simulink model "ALS_Project"  (R2020a)
settings: Solver=FixedStepDiscrete  StartTime=0.0  StopTime=10.0  FixedStep=1  RelTol=1e-3
values from neighbouring files (symbols this model uses):
  Als_mode : value not decoded    [ALS_Project_dd.sldd]
  Carangle = 25.0    [ALS_Project_dd.sldd]    (also in Car_Angle.m = Simulink.Parameter)
  Door_locks : value not decoded    [ALS_Project_dd.sldd]
  Ignition : value not decoded    [ALS_Project_dd.sldd]
  Lanes : value not decoded    [ALS_Project_dd.sldd]
  Lights : value not decoded    [ALS_Project_dd.sldd]
  Obstacles : value not decoded    [ALS_Project_dd.sldd]
  Roads : value not decoded    [ALS_Project_dd.sldd]
  Time = 2.0    [ALS_Project_dd.sldd]    (also in Car_Angle.m = Simulink.Parameter)
  Tunnel : value not decoded    [ALS_Project_dd.sldd]
  Visual : value not decoded    [ALS_Project_dd.sldd]
  Weather : value not decoded    [ALS_Project_dd.sldd]
libraries: simulink x53
settings Model: Creator=hp  LastModifiedBy=hp

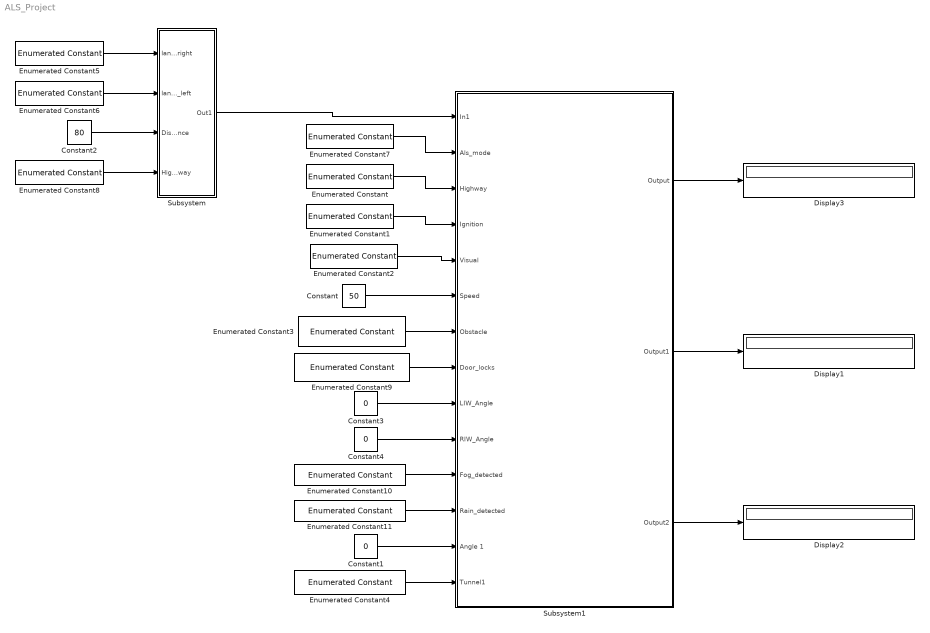
== system ALS_Project ==
  Constant : Constant  Value=50
  Constant1 : Constant  Value=0
  Constant2 : Constant  Value=80
  Constant3 : Constant  Value=0
  Constant4 : Constant  Value=0
  Display1 : Display
  Display2 : Display
  Display3 : Display
  Enumerated Constant : simulink/Sources/Enumerated Constant  OutDataTypeStr=Enum:Roads  Value=Roads.City_road  SampleTime=inf
  Enumerated Constant1 : simulink/Sources/Enumerated Constant  OutDataTypeStr=Enum: Ignition  Value=Ignition.Off  SampleTime=inf
  Enumerated Constant10 : simulink/Sources/Enumerated Constant  OutDataTypeStr=Enum: Weather  Value=Weather.Fog_detected  SampleTime=inf
  Enumerated Constant11 : simulink/Sources/Enumerated Constant  OutDataTypeStr=Enum: Weather  Value=Weather.Rain_detected  SampleTime=inf
  Enumerated Constant2 : simulink/Sources/Enumerated Constant  OutDataTypeStr=Enum: Visual  Value=Visual.Night_mode  SampleTime=inf
  Enumerated Constant3 : simulink/Sources/Enumerated Constant  OutDataTypeStr=Enum: Obstacles  Value=Obstacles.No_Obstacle_detected  SampleTime=inf
  Enumerated Constant4 : simulink/Sources/Enumerated Constant  OutDataTypeStr=Enum: Tunnel  Value=Tunnel.No_Tunnel_detected  SampleTime=inf
  Enumerated Constant5 : simulink/Sources/Enumerated Constant  OutDataTypeStr=Enum: Lanes  Value=Lanes.Lane3_right  SampleTime=inf
  Enumerated Constant6 : simulink/Sources/Enumerated Constant  OutDataTypeStr=Enum: Lanes  Value=Lanes.NoVehicle  SampleTime=inf
  Enumerated Constant7 : simulink/Sources/Enumerated Constant  OutDataTypeStr=Enum: Als_mode  Value=Als_mode.enable  SampleTime=inf
  Enumerated Constant8 : simulink/Sources/Enumerated Constant  OutDataTypeStr=Enum:Roads  Value=Roads.Highway  SampleTime=inf
  Enumerated Constant9 : simulink/Sources/Enumerated Constant  OutDataTypeStr=Enum: Door_locks  Value=Door_locks.Door_locked  SampleTime=inf
  Subsystem : Subsystem  Description=describes about the lanes scenario
  Subsystem1 : Subsystem  Description=normal lightening on highway
  wires:
  Subsystem/1(Out1) -> Subsystem1/1(In1)
  Enumerated Constant/1 -> Subsystem1/3(Highway)
  Enumerated Constant1/1 -> Subsystem1/4(Ignition)
  Enumerated Constant2/1 -> Subsystem1/5(Visual)
  Constant/1 -> Subsystem1/6(Speed)
  Enumerated Constant3/1 -> Subsystem1/7(Obstacle)
  Constant2/1 -> Subsystem/3(Distance)
  Enumerated Constant5/1 -> Subsystem/1(lane1_right)
  Enumerated Constant6/1 -> Subsystem/2(lane1_left)
  Enumerated Constant7/1 -> Subsystem1/2(Als_mode)
  Enumerated Constant8/1 -> Subsystem/4(Highway)
  Enumerated Constant9/1 -> Subsystem1/8(Door_locks)
  Constant4/1 -> Subsystem1/10(RIW_Angle)
  Constant3/1 -> Subsystem1/9(LIW_Angle)
  Constant1/1 -> Subsystem1/13(Angle 1)
  Enumerated Constant4/1 -> Subsystem1/14(Tunnel1)
  Subsystem1/3(Output2) -> Display2/1
  Subsystem1/2(Output1) -> Display1/1
  Subsystem1/1(Output) -> Display3/1
  Enumerated Constant11/1 -> Subsystem1/12(Rain_detected)
  Enumerated Constant10/1 -> Subsystem1/11(Fog_detected)

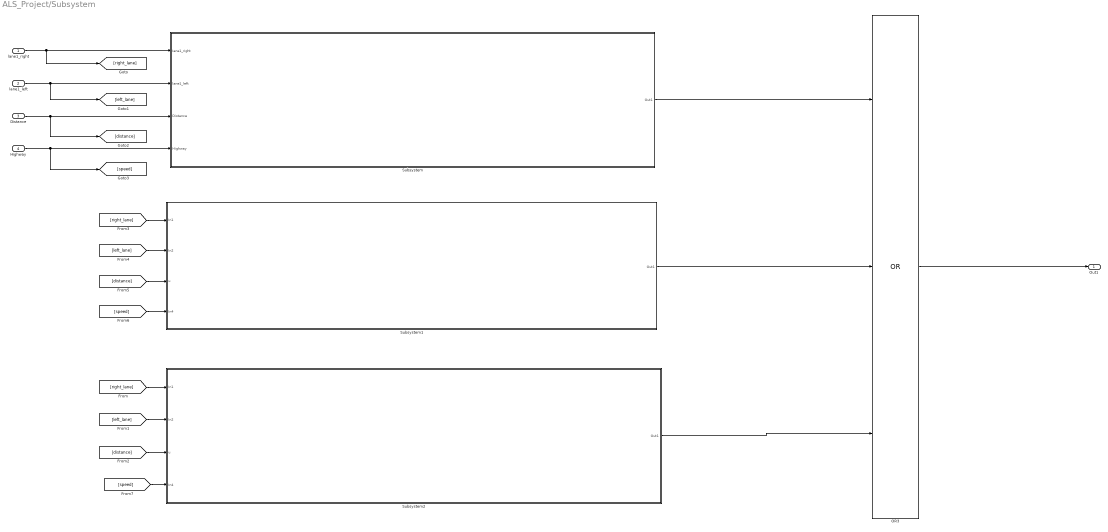
== system ALS_Project/Subsystem ==
  lane1_right : Inport
  lane1_left : Inport  Port=2
  Distance : Inport  Port=3
  Highway : Inport  Port=4
  OR3 : Logic  Operator=OR  Inputs=3  AllPortsSameDT=off  OutDataTypeStr=boolean
  Subsystem : Subsystem  Description=describes about the lane1 scenario
  Subsystem1 : Subsystem  Description=describes about the lane2 scenario
  Subsystem2 : Subsystem  Description=describes about the lane3 scenario
  Out1 : Outport
  wires:
  Highway/1 -> [speed], Subsystem/4(Highway)
  Subsystem1/1(Out1) -> OR3/2
  Subsystem/1(Out1) -> OR3/1
  Subsystem2/1(Out1) -> OR3/3
  lane1_left/1 -> [left_lane], Subsystem/2(lane1_left)
  Distance/1 -> [distance], Subsystem/3(Distance)
  lane1_right/1 -> [right_lane], Subsystem/1(Iane1_right)
  OR3/1 -> Out1/1
  [right_lane] -> Subsystem2/1(In1)
  [left_lane] -> Subsystem2/2(In2)
  [right_lane] -> Subsystem1/1(In1)
  [left_lane] -> Subsystem1/2(In2)
  [distance] -> Subsystem2/3(u)
  [distance] -> Subsystem1/3(u)
  [speed] -> Subsystem1/4(In4)
  [speed] -> Subsystem2/4(In4)

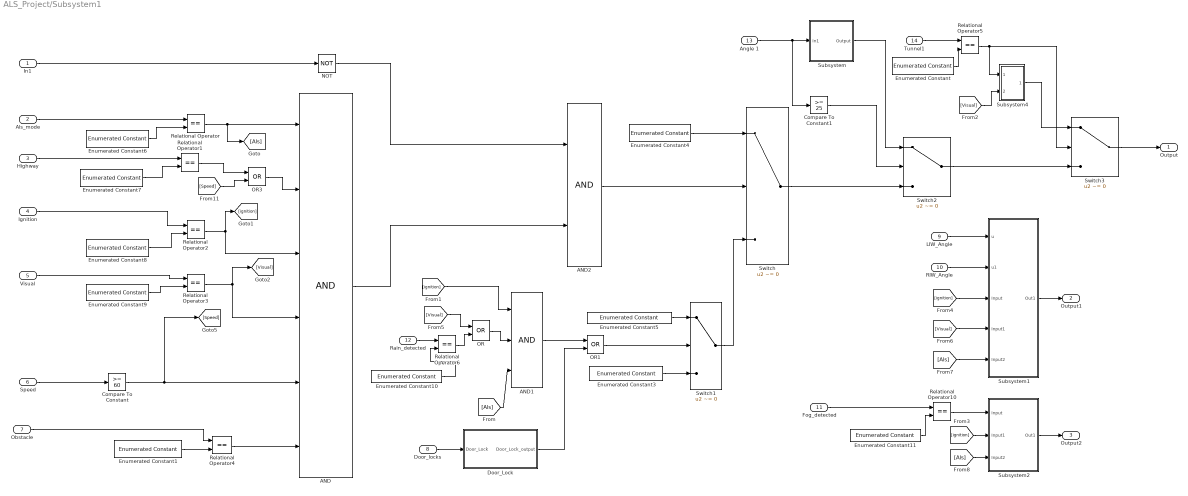
== system ALS_Project/Subsystem1 ==
  In1 : Inport
  Als_mode : Inport  Port=2
  Highway : Inport  Port=3
  Ignition : Inport  Port=4
  Visual : Inport  Port=5
  Speed : Inport  Port=6
  Obstacle : Inport  Port=7
  Door_locks : Inport  Port=8
  LIW_Angle : Inport  Port=9
  RIW_Angle : Inport  Port=10
  Fog_detected : Inport  Port=11
  Rain_detected : Inport  Port=12
  Angle 1 : Inport  Port=13
  Tunnel1 : Inport  Port=14
  AND : Logic  Inputs=6  AllPortsSameDT=off  OutDataTypeStr=boolean
  AND1 : Logic  Inputs=3  AllPortsSameDT=off  OutDataTypeStr=boolean
  AND2 : Logic  AllPortsSameDT=off  OutDataTypeStr=boolean
  Compare To Constant : simulink/Logic and Bit Operations/Compare To Constant  relop=>=  const=60  OutDataTypeStr=boolean
  Compare To Constant1 : simulink/Logic and Bit Operations/Compare To Constant  relop=>=  const=25  OutDataTypeStr=boolean
  Door_Lock : Subsystem
  Enumerated Constant : simulink/Sources/Enumerated Constant  OutDataTypeStr=Enum: Tunnel  Value=Tunnel.Tunnel_detected  SampleTime=inf
  Enumerated Constant1 : simulink/Sources/Enumerated Constant  OutDataTypeStr=Enum:Obstacles  Value=Obstacles.No_Obstacle_detected  SampleTime=inf
  Enumerated Constant10 : simulink/Sources/Enumerated Constant  OutDataTypeStr=Enum: Weather  Value=Weather.Rain_detected  SampleTime=inf
  Enumerated Constant11 : simulink/Sources/Enumerated Constant  OutDataTypeStr=Enum: Weather  Value=Weather.Fog_detected  SampleTime=inf
  Enumerated Constant3 : simulink/Sources/Enumerated Constant  OutDataTypeStr=Enum: Lights  Value=Lights.Headlights_Off  SampleTime=inf
  Enumerated Constant4 : simulink/Sources/Enumerated Constant  OutDataTypeStr=Enum: Lights  Value=Lights.High_Beam  SampleTime=inf
  Enumerated Constant5 : simulink/Sources/Enumerated Constant  OutDataTypeStr=Enum: Lights  Value=Lights.Low_Beam  SampleTime=inf
  Enumerated Constant6 : simulink/Sources/Enumerated Constant  OutDataTypeStr=Enum: Als_mode  Value=Als_mode.enable  SampleTime=inf
  Enumerated Constant7 : simulink/Sources/Enumerated Constant  OutDataTypeStr=Enum: Roads  Value=Roads.Highway  SampleTime=inf
  Enumerated Constant8 : simulink/Sources/Enumerated Constant  OutDataTypeStr=Enum: Ignition  Value=Ignition.On  SampleTime=inf
  Enumerated Constant9 : simulink/Sources/Enumerated Constant  OutDataTypeStr=Enum: Visual  Value=Visual.Night_mode  SampleTime=inf
  NOT : Logic  Operator=NOT  IconShape=distinctive  AllPortsSameDT=off  OutDataTypeStr=boolean
  OR : Logic  Operator=OR  AllPortsSameDT=off  OutDataTypeStr=boolean
  OR1 : Logic  Operator=OR  AllPortsSameDT=off  OutDataTypeStr=boolean
  OR3 : Logic  Operator=OR  AllPortsSameDT=off  OutDataTypeStr=boolean
  Relational Operator{,1..6,10} (8 alike) : RelationalOperator  Operator===  OutDataTypeStr=boolean  RndMeth=Simplest
  Subsystem : Subsystem
  Subsystem1 : Subsystem
  Subsystem2 : Subsystem
  Subsystem4 : Subsystem
  Switch{,1..3} (4 alike) : Switch  Criteria=u2 ~= 0
  Output : Outport
  Output1 : Outport  Port=2
  Output2 : Outport  Port=3
  wires:
  Relational Operator3/1 -> [Visual], AND/4
  Relational Operator/1 -> [Als], AND/1
  Relational Operator2/1 -> [ignition], AND/3
  Enumerated Constant7/1 -> Relational Operator1/2
  Switch1/1 -> Switch/3
  Enumerated Constant9/1 -> Relational Operator3/2
  Als_mode/1 -> Relational Operator/1
  Highway/1 -> Relational Operator1/1
  Enumerated Constant8/1 -> Relational Operator2/2
  Enumerated Constant5/1 -> Switch1/1
  Ignition/1 -> Relational Operator2/1
  Visual/1 -> Relational Operator3/1
  Enumerated Constant4/1 -> Switch/1
  In1/1 -> NOT/1
  Enumerated Constant6/1 -> Relational Operator/2
  NOT/1 -> AND2/1
  [ignition] -> AND1/1
  Obstacle/1 -> Relational Operator4/1
  Enumerated Constant1/1 -> Relational Operator4/2
  Relational Operator4/1 -> AND/6
  [Visual] -> OR/1
  OR/1 -> AND1/2
  Enumerated Constant3/1 -> Switch1/3
  AND/1 -> AND2/2
  AND2/1 -> Switch/2
  RIW_Angle/1 -> Subsystem1/2(u1)
  LIW_Angle/1 -> Subsystem1/1(u)
  Subsystem1/1(Out1) -> Output1/1
  Subsystem2/1(Out1) -> Output2/1
  Fog_detected/1 -> Relational Operator10/1
  Enumerated Constant11/1 -> Relational Operator10/2
  [ignition] -> Subsystem1/3(Input)
  [Visual] -> Subsystem1/4(Input1)
  [Als] -> Subsystem1/5(Input2)
  Relational Operator10/1 -> Subsystem2/1(Input)
  [ignition] -> Subsystem2/2(Input1)
  [Als] -> Subsystem2/3(Input2)
  OR1/1 -> Switch1/2
  AND1/1 -> OR1/1
  Rain_detected/1 -> Relational Operator6/1
  Enumerated Constant10/1 -> Relational Operator6/2
  [Als] -> AND1/3
  Speed/1 -> Compare To Constant/1
  Compare To Constant/1 -> [Speed], AND/5
  OR3/1 -> AND/2
  Relational Operator1/1 -> OR3/1
  [Speed] -> OR3/2
  Door_locks/1 -> Door_Lock/1(Door_Lock)
  Door_Lock/1(Door_Lock_output) -> OR1/2
  Angle 1/1 -> Compare To Constant1/1, Subsystem/1(In1)
  Switch/1 -> Switch2/3
  Subsystem/1(Output) -> Switch2/1
  Compare To Constant1/1 -> Switch2/2
  Switch3/1 -> Output/1
  Switch2/1 -> Switch3/3
  Relational Operator6/1 -> OR/2
  Relational Operator5/1 -> Switch3/2, Subsystem4/1(In1)
  Tunnel1/1 -> Relational Operator5/1
  Enumerated Constant/1 -> Relational Operator5/2
  Subsystem4/1(Output) -> Switch3/1
  [Visual] -> Subsystem4/2(In2)

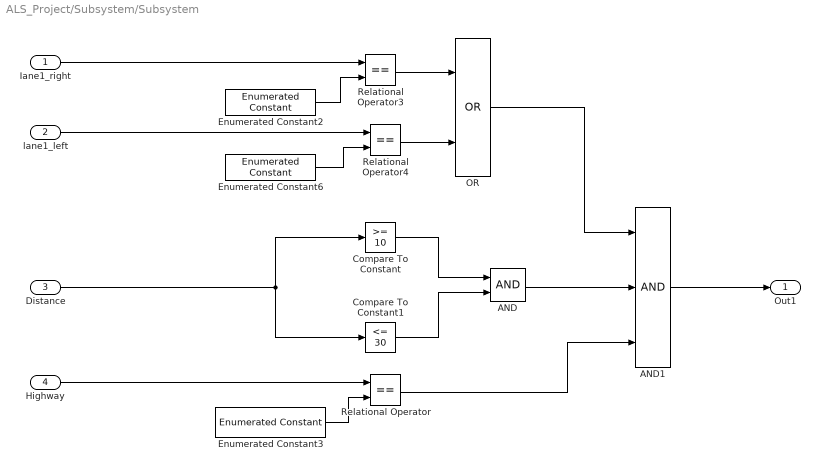
== system ALS_Project/Subsystem/Subsystem ==
  Iane1_right : Inport
  lane1_left : Inport  Port=2
  Distance : Inport  Port=3
  Highway : Inport  Port=4
  AND : Logic  AllPortsSameDT=off  OutDataTypeStr=boolean
  AND1 : Logic  Inputs=3  AllPortsSameDT=off  OutDataTypeStr=boolean
  Compare To Constant : simulink/Logic and Bit Operations/Compare To Constant  relop=>=  const=10  OutDataTypeStr=boolean
  Compare To Constant1 : simulink/Logic and Bit Operations/Compare To Constant  relop=<=  const=30  OutDataTypeStr=boolean
  Enumerated Constant2 : simulink/Sources/Enumerated Constant  OutDataTypeStr=Enum: Lanes  Value=Lanes.Lane1_right  SampleTime=inf
  Enumerated Constant3 : simulink/Sources/Enumerated Constant  OutDataTypeStr=Enum:Roads  Value=Roads.Highway  SampleTime=inf
  Enumerated Constant6 : simulink/Sources/Enumerated Constant  OutDataTypeStr=Enum: Lanes  Value=Lanes.Lane1_left  SampleTime=inf
  OR : Logic  Operator=OR  AllPortsSameDT=off  OutDataTypeStr=boolean
  Relational Operator : RelationalOperator  Operator===  OutDataTypeStr=boolean  RndMeth=Simplest
  Relational Operator3 : RelationalOperator  Operator===  OutDataTypeStr=boolean  RndMeth=Simplest
  Relational Operator4 : RelationalOperator  Operator===  OutDataTypeStr=boolean  RndMeth=Simplest
  Out1 : Outport
  wires:
  Enumerated Constant6/1 -> Relational Operator4/2
  Relational Operator3/1 -> OR/1
  Compare To Constant/1 -> AND/1
  OR/1 -> AND1/1
  Distance/1 -> Compare To Constant/1, Compare To Constant1/1
  Relational Operator/1 -> AND1/3
  Highway/1 -> Relational Operator/1
  Enumerated Constant2/1 -> Relational Operator3/2
  lane1_left/1 -> Relational Operator4/1
  Enumerated Constant3/1 -> Relational Operator/2
  AND/1 -> AND1/2
  Compare To Constant1/1 -> AND/2
  Relational Operator4/1 -> OR/2
  Iane1_right/1 -> Relational Operator3/1
  AND1/1 -> Out1/1

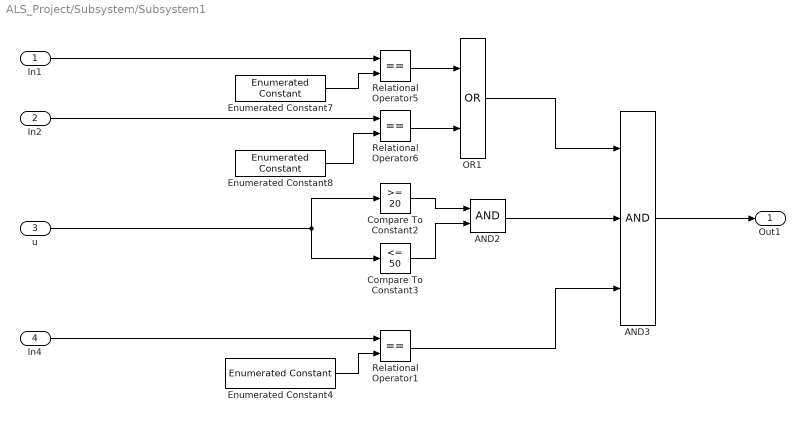
== system ALS_Project/Subsystem/Subsystem1 ==
  In1 : Inport
  In2 : Inport  Port=2
  u : Inport  Port=3
  In4 : Inport  Port=4
  AND2 : Logic  AllPortsSameDT=off  OutDataTypeStr=boolean
  AND3 : Logic  Inputs=3  AllPortsSameDT=off  OutDataTypeStr=boolean
  Compare To Constant2 : simulink/Logic and Bit Operations/Compare To Constant  relop=>=  const=20  OutDataTypeStr=boolean
  Compare To Constant3 : simulink/Logic and Bit Operations/Compare To Constant  relop=<=  const=50  OutDataTypeStr=boolean
  Enumerated Constant4 : simulink/Sources/Enumerated Constant  OutDataTypeStr=Enum:Roads  Value=Roads.Highway  SampleTime=inf
  Enumerated Constant7 : simulink/Sources/Enumerated Constant  OutDataTypeStr=Enum: Lanes  Value=Lanes.Lane2_right  SampleTime=inf
  Enumerated Constant8 : simulink/Sources/Enumerated Constant  OutDataTypeStr=Enum: Lanes  Value=Lanes.Lane2_left  SampleTime=inf
  OR1 : Logic  Operator=OR  AllPortsSameDT=off  OutDataTypeStr=boolean
  Relational Operator1 : RelationalOperator  Operator===  OutDataTypeStr=boolean  RndMeth=Simplest
  Relational Operator5 : RelationalOperator  Operator===  OutDataTypeStr=boolean  RndMeth=Simplest
  Relational Operator6 : RelationalOperator  Operator===  OutDataTypeStr=boolean  RndMeth=Simplest
  Out1 : Outport
  wires:
  u/1 -> Compare To Constant2/1, Compare To Constant3/1
  AND3/1 -> Out1/1
  In2/1 -> Relational Operator6/1
  Enumerated Constant4/1 -> Relational Operator1/2
  Relational Operator1/1 -> AND3/3
  Compare To Constant3/1 -> AND2/2
  Enumerated Constant7/1 -> Relational Operator5/2
  OR1/1 -> AND3/1
  Compare To Constant2/1 -> AND2/1
  AND2/1 -> AND3/2
  In4/1 -> Relational Operator1/1
  Enumerated Constant8/1 -> Relational Operator6/2
  Relational Operator6/1 -> OR1/2
  Relational Operator5/1 -> OR1/1
  In1/1 -> Relational Operator5/1

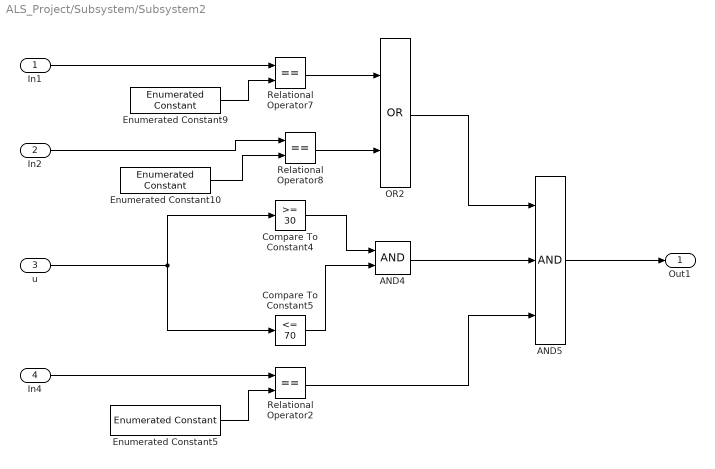
== system ALS_Project/Subsystem/Subsystem2 ==
  In1 : Inport
  In2 : Inport  Port=2
  u : Inport  Port=3
  In4 : Inport  Port=4
  AND4 : Logic  AllPortsSameDT=off  OutDataTypeStr=boolean
  AND5 : Logic  Inputs=3  AllPortsSameDT=off  OutDataTypeStr=boolean
  Compare To Constant4 : simulink/Logic and Bit Operations/Compare To Constant  relop=>=  const=30  OutDataTypeStr=boolean
  Compare To Constant5 : simulink/Logic and Bit Operations/Compare To Constant  relop=<=  const=70  OutDataTypeStr=boolean
  Enumerated Constant10 : simulink/Sources/Enumerated Constant  OutDataTypeStr=Enum: Lanes  Value=Lanes.Lane3_left  SampleTime=inf
  Enumerated Constant5 : simulink/Sources/Enumerated Constant  OutDataTypeStr=Enum:Roads  Value=Roads.Highway  SampleTime=inf
  Enumerated Constant9 : simulink/Sources/Enumerated Constant  OutDataTypeStr=Enum: Lanes  Value=Lanes.Lane3_right  SampleTime=inf
  OR2 : Logic  Operator=OR  AllPortsSameDT=off  OutDataTypeStr=boolean
  Relational Operator2 : RelationalOperator  Operator===  OutDataTypeStr=boolean  RndMeth=Simplest
  Relational Operator7 : RelationalOperator  Operator===  OutDataTypeStr=boolean  RndMeth=Simplest
  Relational Operator8 : RelationalOperator  Operator===  OutDataTypeStr=boolean  RndMeth=Simplest
  Out1 : Outport
  wires:
  u/1 -> Compare To Constant4/1, Compare To Constant5/1
  Relational Operator8/1 -> OR2/2
  AND5/1 -> Out1/1
  In4/1 -> Relational Operator2/1
  Relational Operator7/1 -> OR2/1
  Compare To Constant5/1 -> AND4/2
  Relational Operator2/1 -> AND5/3
  OR2/1 -> AND5/1
  Enumerated Constant5/1 -> Relational Operator2/2
  Compare To Constant4/1 -> AND4/1
  AND4/1 -> AND5/2
  Enumerated Constant9/1 -> Relational Operator7/2
  Enumerated Constant10/1 -> Relational Operator8/2
  In2/1 -> Relational Operator8/1
  In1/1 -> Relational Operator7/1

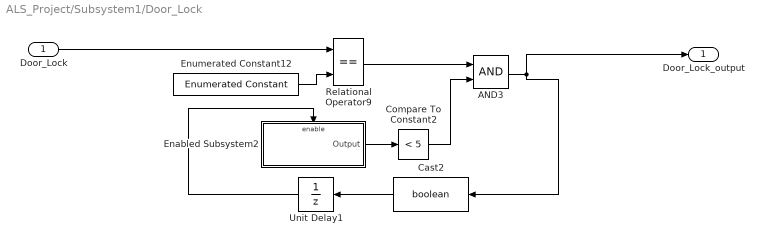
== system ALS_Project/Subsystem1/Door_Lock ==
  Door_Lock : Inport
  AND3 : Logic  AllPortsSameDT=off  OutDataTypeStr=boolean
  Cast2 : DataTypeConversion  OutDataTypeStr=boolean
  Compare To Constant2 : simulink/Logic and Bit Operations/Compare To Constant  relop=<  const=5  OutDataTypeStr=boolean
  Enabled Subsystem2 : Subsystem  TreatAsAtomicUnit=on
  Enumerated Constant12 : simulink/Sources/Enumerated Constant  OutDataTypeStr=Enum: Door_locks  Value=Door_locks.Door_locked  SampleTime=inf
  Relational Operator9 : RelationalOperator  Operator===  OutDataTypeStr=boolean  RndMeth=Simplest
  Unit Delay1 : UnitDelay  SampleTime=-1  HasFrameUpgradeWarning=on
  Door_Lock_output : Outport
  wires:
  Relational Operator9/1 -> AND3/1
  Cast2/1 -> Unit Delay1/1
  Compare To Constant2/1 -> AND3/2
  AND3/1 -> Cast2/1, Door_Lock_output/1
  Enabled Subsystem2/1(Output) -> Compare To Constant2/1
  Enumerated Constant12/1 -> Relational Operator9/2
  Unit Delay1/1 -> Enabled Subsystem2/Enable
  Door_Lock/1 -> Relational Operator9/1

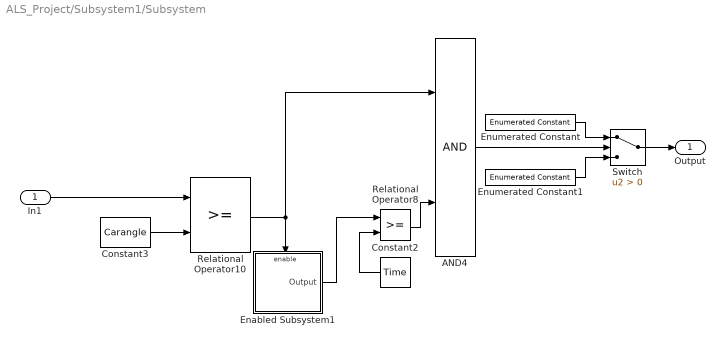
== system ALS_Project/Subsystem1/Subsystem ==
  In1 : Inport
  AND4 : Logic  AllPortsSameDT=off  OutDataTypeStr=boolean
  Constant2 : Constant  Value=Time
  Constant3 : Constant  Value=Carangle
  Enabled Subsystem1 : Subsystem  TreatAsAtomicUnit=on
  Enumerated Constant : simulink/Sources/Enumerated Constant  OutDataTypeStr=Enum: Lights  Value=Lights.High_Beam  SampleTime=inf
  Enumerated Constant1 : simulink/Sources/Enumerated Constant  OutDataTypeStr=Enum: Lights  Value=Lights.Low_Beam  SampleTime=inf
  Relational Operator10 : RelationalOperator  OutDataTypeStr=boolean  RndMeth=Simplest
  Relational Operator8 : RelationalOperator  OutDataTypeStr=boolean  RndMeth=Simplest
  Switch : Switch  Criteria=u2 > Threshold
  Output : Outport
  wires:
  In1/1 -> Relational Operator10/1
  Constant3/1 -> Relational Operator10/2
  Enabled Subsystem1/1(Output) -> Relational Operator8/1
  Constant2/1 -> Relational Operator8/2
  Relational Operator10/1 -> AND4/1, Enabled Subsystem1/Enable
  Relational Operator8/1 -> AND4/2
  AND4/1 -> Switch/2
  Switch/1 -> Output/1
  Enumerated Constant/1 -> Switch/1
  Enumerated Constant1/1 -> Switch/3

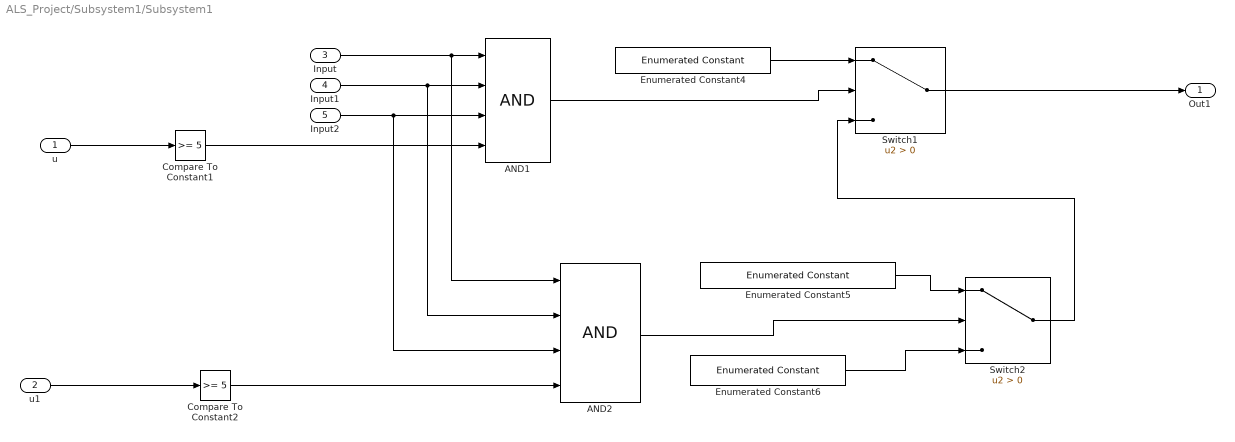
== system ALS_Project/Subsystem1/Subsystem1 ==
  u : Inport
  u1 : Inport  Port=2
  Input : Inport  Port=3
  Input1 : Inport  Port=4
  Input2 : Inport  Port=5
  AND1 : Logic  Inputs=4  AllPortsSameDT=off  OutDataTypeStr=boolean
  AND2 : Logic  Inputs=4  AllPortsSameDT=off  OutDataTypeStr=boolean
  Compare To Constant1 : simulink/Logic and Bit Operations/Compare To Constant  relop=>=  const=5  OutDataTypeStr=boolean
  Compare To Constant2 : simulink/Logic and Bit Operations/Compare To Constant  relop=>=  const=5  OutDataTypeStr=boolean
  Enumerated Constant4 : simulink/Sources/Enumerated Constant  OutDataTypeStr=Enum: Lights  Value=Lights.Left_Corner_Light_On  SampleTime=inf
  Enumerated Constant5 : simulink/Sources/Enumerated Constant  OutDataTypeStr=Enum: Lights  Value=Lights.Right_Corner_Light_On  SampleTime=inf
  Enumerated Constant6 : simulink/Sources/Enumerated Constant  OutDataTypeStr=Enum: Lights  Value=Lights.Corner_Light_Off  SampleTime=inf
  Switch1 : Switch  Criteria=u2 > Threshold
  Switch2 : Switch  Criteria=u2 > Threshold
  Out1 : Outport
  wires:
  Switch2/1 -> Switch1/3
  Compare To Constant1/1 -> AND1/4
  Enumerated Constant5/1 -> Switch2/1
  Enumerated Constant6/1 -> Switch2/3
  Compare To Constant2/1 -> AND2/4
  Enumerated Constant4/1 -> Switch1/1
  AND2/1 -> Switch2/2
  Switch1/1 -> Out1/1
  u/1 -> Compare To Constant1/1
  AND1/1 -> Switch1/2
  u1/1 -> Compare To Constant2/1
  Input/1 -> AND2/1, AND1/1
  Input1/1 -> AND2/2, AND1/2
  Input2/1 -> AND2/3, AND1/3

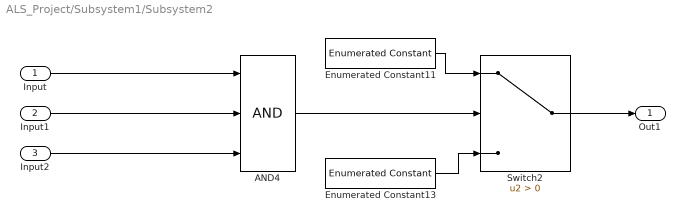
== system ALS_Project/Subsystem1/Subsystem2 ==
  Input : Inport
  Input1 : Inport  Port=2
  Input2 : Inport  Port=3
  AND4 : Logic  Inputs=3  AllPortsSameDT=off  OutDataTypeStr=boolean
  Enumerated Constant11 : simulink/Sources/Enumerated Constant  OutDataTypeStr=Enum:Lights  Value=Lights.Fog_light_On  SampleTime=inf
  Enumerated Constant13 : simulink/Sources/Enumerated Constant  OutDataTypeStr=Enum:Lights  Value=Lights.Fog_light_Off  SampleTime=inf
  Switch2 : Switch  Criteria=u2 > Threshold
  Out1 : Outport
  wires:
  AND4/1 -> Switch2/2
  Switch2/1 -> Out1/1
  Enumerated Constant13/1 -> Switch2/3
  Enumerated Constant11/1 -> Switch2/1
  Input/1 -> AND4/1
  Input1/1 -> AND4/2
  Input2/1 -> AND4/3

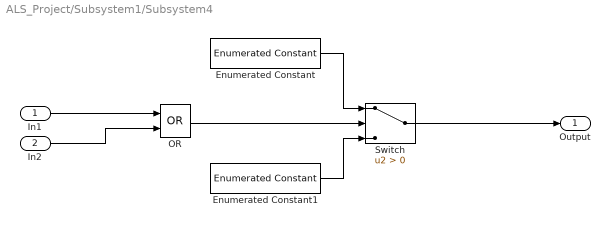
== system ALS_Project/Subsystem1/Subsystem4 ==
  In1 : Inport
  In2 : Inport  Port=2
  Enumerated Constant : simulink/Sources/Enumerated Constant  OutDataTypeStr=Enum: Lights  Value=Lights.High_Beam  SampleTime=inf
  Enumerated Constant1 : simulink/Sources/Enumerated Constant  OutDataTypeStr=Enum: Lights  Value=Lights.Low_Beam  SampleTime=inf
  OR : Logic  Operator=OR  AllPortsSameDT=off  OutDataTypeStr=boolean
  Switch : Switch  Criteria=u2 > Threshold
  Output : Outport
  wires:
  Enumerated Constant/1 -> Switch/1
  Enumerated Constant1/1 -> Switch/3
  Switch/1 -> Output/1
  OR/1 -> Switch/2
  In1/1 -> OR/1
  In2/1 -> OR/2

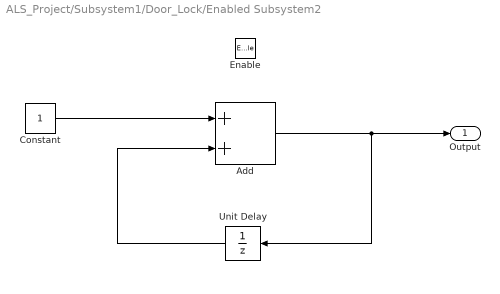
== system ALS_Project/Subsystem1/Door_Lock/Enabled Subsystem2 ==
  Enable : EnablePort
  Add : Sum
  Constant : Constant
  Unit Delay : UnitDelay  SampleTime=-1  HasFrameUpgradeWarning=on
  Output : Outport  VectorParamsAs1DForOutWhenUnconnected=off
  wires:
  Add/1 -> Output/1, Unit Delay/1
  Constant/1 -> Add/1
  Unit Delay/1 -> Add/2

== system ALS_Project/Subsystem1/Subsystem/Enabled Subsystem1 ==
  Enable : EnablePort  StatesWhenEnabling=reset
  Add : Sum
  Constant : Constant
  Unit Delay : UnitDelay  SampleTime=-1  HasFrameUpgradeWarning=on
  Output : Outport  OutputWhenDisabled=reset  InitialOutput=[0]
  wires:
  Constant/1 -> Add/1
  Add/1 -> Unit Delay/1, Output/1
  Unit Delay/1 -> Add/2
